simulink model "unsigned2signed"  (Simulink 7.7)
settings: Solver=ode45  StartTime=0.0  StopTime=10.0  RelTol=1e-3
libraries: xbsIndex_r4 x4
settings Model: Creator=Lerwys  LastModifiedBy=Lerwys

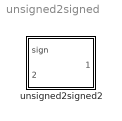
== system unsigned2signed ==
  unsigned2signed2 : Subsystem

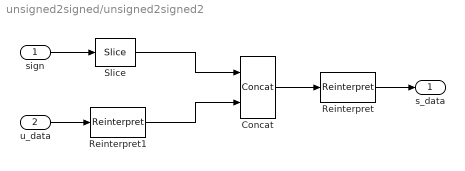
== system unsigned2signed/unsigned2signed2 ==
  sign : Inport
  u_data : Inport  Port=2
  Concat : xbsIndex_r4/Concat  num_inputs=2  dbl_ovrd=off  block_type=concat
  Reinterpret : xbsIndex_r4/Reinterpret  force_arith_type=on  arith_type="Signed  (2's comp)"  force_bin_pt=on  bin_pt=22  block_type=reinterpret
  Reinterpret1 : xbsIndex_r4/Reinterpret  force_arith_type=off  arith_type="Signed  (2's comp)"  force_bin_pt=on  bin_pt=0  block_type=reinterpret
  Slice : xbsIndex_r4/Slice  nbits=1  boolean_output=off  mode=Upper Bit Location + Width  bit1=0  base1=MSB of Input  bit0=0  base0=LSB of Input  dbl_ovrd=off  block_type=slice
  s_data : Outport
  wires:
  Concat/1 -> Reinterpret/1
  Slice/1 -> Concat/1
  sign/1 -> Slice/1
  Reinterpret/1 -> s_data/1
  u_data/1 -> Reinterpret1/1
  Reinterpret1/1 -> Concat/2
